simulink model "flatball_hummel_mdl_validation_IC"  (R2021b)
settings: Solver=ode1be  StartTime=0.0  StopTime=30  FixedStep=0.001  MaxStep=0.01  MinStep=0.01  RelTol=1e-3
values from neighbouring files (symbols this model uses):
  amb = evalin( 'base', 'amb')    [flatball_6dof_eqom.m]
  disc = evalin( 'base', 'disc')    [flatball_6dof_eqom.m]    (also in flatball_6dof_init.m = struct; flatball_init_disc_params.m = struct)
  k_launch_F_t_release = 0.60    (= 0.6)    [flatball_6dof_hucker_init.m]
  k_launch_Fx_kd = 2e-2    (= 0.02)    [flatball_6dof_hucker_init.m]
  k_launch_Fx_ki = 15    [flatball_6dof_hucker_init.m]
  k_launch_Fx_kp = 7.5    [flatball_6dof_hucker_init.m]
  k_launch_Fx_sat_hi = 150    [flatball_6dof_hucker_init.m]
  k_launch_Fx_sat_lo = -150    [flatball_6dof_hucker_init.m]
  k_launch_Fx_t_launch_begin = 0.50    (= 0.5)    [flatball_6dof_hucker_init.m]
  k_launch_Fx_t_launch_end = k_launch_F_t_release    (= 0.6)    [flatball_6dof_hucker_init.m]
  k_launch_Fx_tau = 1e-2    (= 0.01)    [flatball_6dof_hucker_init.m]
  k_launch_Fy_kd = k_launch_Fx_kd    (= 0.02)    [flatball_6dof_hucker_init.m]
  k_launch_Fy_ki = k_launch_Fx_ki    (= 15)    [flatball_6dof_hucker_init.m]
  k_launch_Fy_kp = k_launch_Fx_kp    (= 7.5)    [flatball_6dof_hucker_init.m]
  k_launch_Fy_sat_hi = k_launch_Fx_sat_hi    (= 150)    [flatball_6dof_hucker_init.m]
  k_launch_Fy_sat_lo = k_launch_Fx_sat_lo    (= -150)    [flatball_6dof_hucker_init.m]
  k_launch_Fy_t_launch_begin = 0.50    (= 0.5)    [flatball_6dof_hucker_init.m]
  k_launch_Fy_t_launch_end = k_launch_F_t_release    (= 0.6)    [flatball_6dof_hucker_init.m]
  k_launch_Fy_tau = 1e-2    (= 0.01)    [flatball_6dof_hucker_init.m]
  k_launch_Fz_kd = 2.5    [flatball_6dof_hucker_init.m]
  k_launch_Fz_ki = 50    [flatball_6dof_hucker_init.m]
  k_launch_Fz_kp = 20    [flatball_6dof_hucker_init.m]
  k_launch_Fz_sat_hi = 25    [flatball_6dof_hucker_init.m]
  k_launch_Fz_sat_lo = -25    [flatball_6dof_hucker_init.m]
  k_launch_Fz_t_launch_begin = 0.10    (= 0.1)    [flatball_6dof_hucker_init.m]
  k_launch_Fz_t_launch_end = k_launch_F_t_release    (= 0.6)    [flatball_6dof_hucker_init.m]
  k_launch_Fz_tau = 1e-2    (= 0.01)    [flatball_6dof_hucker_init.m]
  k_launch_M_t_release = 0.60    (= 0.6)    [flatball_6dof_hucker_init.m]
  k_launch_Mx_kd = 0.125    [flatball_6dof_hucker_init.m]
  k_launch_Mx_ki = 1.125    [flatball_6dof_hucker_init.m]
  k_launch_Mx_kp = 3.5    [flatball_6dof_hucker_init.m]
  k_launch_Mx_sat_hi = 2.5    [flatball_6dof_hucker_init.m]
  k_launch_Mx_sat_lo = -2.5    [flatball_6dof_hucker_init.m]
  k_launch_Mx_t_launch_begin = 0.30    (= 0.3)    [flatball_6dof_hucker_init.m]
  k_launch_Mx_t_launch_end = k_launch_M_t_release    (= 0.6)    [flatball_6dof_hucker_init.m]
  k_launch_Mx_tau = 1e-2    (= 0.01)    [flatball_6dof_hucker_init.m]
  k_launch_My_kd = 0.1125    [flatball_6dof_hucker_init.m]
  k_launch_My_ki = 5.5    [flatball_6dof_hucker_init.m]
  k_launch_My_kp = 4.25    [flatball_6dof_hucker_init.m]
  k_launch_My_sat_hi = 2.5    [flatball_6dof_hucker_init.m]
  k_launch_My_sat_lo = -2.5    [flatball_6dof_hucker_init.m]
  k_launch_My_t_launch_begin = 0.40    (= 0.4)    [flatball_6dof_hucker_init.m]
  k_launch_My_t_launch_end = k_launch_M_t_release    (= 0.6)    [flatball_6dof_hucker_init.m]
  k_launch_My_tau = 1e-2    (= 0.01)    [flatball_6dof_hucker_init.m]
  k_launch_Mz_kd = 1e-8    (= 1e-08)    [flatball_6dof_hucker_init.m]
  k_launch_Mz_ki = 0.2575    [flatball_6dof_hucker_init.m]
  k_launch_Mz_kp = 0.25    [flatball_6dof_hucker_init.m]
  k_launch_Mz_sat_hi = 7.5    [flatball_6dof_hucker_init.m]
  k_launch_Mz_sat_lo = -7.5    [flatball_6dof_hucker_init.m]
  k_launch_Mz_t_launch_begin = 0.20    (= 0.2)    [flatball_6dof_hucker_init.m]
  k_launch_Mz_t_launch_end = k_launch_M_t_release    (= 0.6)    [flatball_6dof_hucker_init.m]
  k_launch_Mz_tau = 1e-2    (= 0.01)    [flatball_6dof_hucker_init.m]
  X0_crowther_f2302 = [      -0.90 -0.63 -0.91,  4.48 12.52 1.84,      -0.07 0.21 5.03,    -26.25 -5.19 52.85]    [hummel_thesis_mdl_validation.m]
  X0_desired = X0_crowther_f2302    [hummel_thesis_mdl_validation.m]
  X0_hummel_f2302 = [      -0.90 -0.63 -0.91,  13.42 -0.41 0.001,      -0.07 0.21 5.03,    -14.94 -1.48 54.25]    [hummel_thesis_mdl_validation.m]
libraries: slpidlib x6, simulink x2, aerolibanim x2, aerolibnav x2, matrix_library x2, mspfiltlib x1
(part 3 of 3)

== matlab function flatball_hummel_mdl_validation_IC/calc-M/q-inf/vector-norm ==
  data: vec input; norm output
function norm = fcn( vec)

norm = sqrt( vec(1)*vec(1) + vec(2)*vec(2) + vec(3)*vec(3));

== matlab function flatball_hummel_mdl_validation_IC/rotations/X-to-T_c_N ==
  data: X input; T_c_N output
function T_c_N  = f( X)
%% internal states
phi = X(7); theta = X(8);

%% helper variables
sin_theta = sin( theta);
cos_theta = cos( theta);
sin_phi = sin( phi);
cos_phi = cos(phi);

T_c_N = [
    cos_theta sin_theta*sin_phi -sin_theta*cos_phi;
    0 cos_phi sin_phi;
    sin_theta -cos_theta*sin_phi cos_theta*cos_phi
    ];

== matlab function flatball_hummel_mdl_validation_IC/lab/helpers/Subsystem1/transformation-matrices/Ta ==
  data: TH input; M output
function M  = Ta( TH)
% transformation matrix
%
phi = TH(1); theta = TH(2); psi = TH(3);

cos_theta = cos( theta);
cos_phi = cos( phi);
cos_psi = cos( psi);
sin_phi = sin( phi);
sin_theta = sin( theta);
sin_psi = sin( psi);

M = [ ...
    cos_theta*cos_psi sin_phi*sin_theta*cos_phi-cos_phi*sin_psi cos_phi*sin_theta*cos_psi+sin_phi*sin_psi;
    cos_theta*sin_psi sin_phi*sin_theta*sin_psi+cos_phi*cos_psi cos_phi*sin_theta*sin_psi-sin_phi*cos_psi;
    -sin_theta sin_phi*cos_theta cos_phi*cos_theta
    ];

% tan_theta = tan( theta);
% sec_theta = sec( theta);
% transform_r_phi_thea_psi = [
%     1 sin_phi*tan_theta cos_phi*tan_theta
%     0 cos_phi -sin_phi
%     0 sin_phi*sec_theta cos_phi*sec_theta
%     ];

== matlab function flatball_hummel_mdl_validation_IC/rotations/X-to-wD_N_inC ==
  data: X input; wD_N_inC output
function wD_N_inC  = f( X)
%% internal states
theta = X(8);
phidot = X(10); thetadot = X(11); gammadot = X(12);

%% helper variables
sin_theta = sin( theta);
cos_theta = cos( theta);

wD_N_inC = [phidot*cos_theta thetadot phidot*sin_theta+gammadot];

== matlab function flatball_hummel_mdl_validation_IC/lab/wrk/flatball_6dof ==
  data: X input; Xdot output; lift output; drag output; alpha output; AdvR output; E_trans output; E_rot output
function [Xdot, lift, drag, alpha, AdvR, E_trans, E_rot]  = flatball_6dof_eom( X)
% flatball equations of motion - NED (north-east-down) configuration
%

%% internal states
x = X(1); y = X(2); z = X(3);
xdot = X(4); ydot = X(5); zdot = X(6);

phi = X(7); theta = X(8); gamma = X(9);
phidot = X(10); thetadot = X(11); gammadot = X(12);

Xdot = zeros(1,12);

%% define ambient parameters
amb.g = 9.81; % m/s^2
amb.rho = 1.23; % Kg/m^3

%% define non-aerodynamic parameters
disc = struct;
disc.m = 0.175; % Kg
disc.A = 0.057; % m^2
disc.d = 2*sqrt(0.057/pi); % 2*sqrt(disc.A/pi); % diameter
disc.Ia = 0.002352; % moment of inertia about the spinning axis
disc.Id = 0.001219; % moment of inertia about the planar axis'

disc.alpha0 = -4 * pi/180.0;

%% THE THREE ESTIMATED COEFFICIENTS
disc.CMq= -1.44E-02;
disc.CRp =-1.25E-02;
disc.CNr = -3.41E-05; % long flight f2302

%% THE seven COEFFICIENTS estimated from three flights
disc.CL0= 0.3331;
disc.CLa= 1.9124;
disc.CD0= 0.1769;
disc.CDa= 0.685;
disc.CM0= -0.0821;
disc.CMa= 0.4338;
disc.CRr= 0.00171; % for nondimensionalization = sqrt(d/g), magnitude of CRr changes

%% CL =[ rad CL deg]
disc.CL_data=[ -0.1745 -0.2250 -10; ...
-0.05236 0 -3; ...
0 0.150 0; ...
0.08727 0.4500 5; ...
0.17453 0.7250 10; ...
0.26180 0.9750 15; ...
0.34907 1.2000 20; ...
0.43633 1.4500 25; ...
0.52360 1.6750 30];

%% CD =[ rad CD deg]
disc.CD_data=[ -0.1745 0.1500 -10; ...
-0.05236 0.0800 -3; ...
0 0.1000 0; ...
0.08727 0.1500 5; ...
0.1745 0.2600 10; ...
0.26180 0.3900 15; ...
0.3491 0.5700 20; ...
0.4363 0.7500 25; ...
0.5236 0.9200 30];

%% CM =[ rad CM deg]
disc.CM_data=[-0.174532925 -0.0380 -10; ...
-0.087266463 -0.0220 -5; ...
-0.052359878 -0.0140 -3; ...
0 -0.0060 0; ...
0.052359878 -0.0060 3; ...
0.104719755 -0.0020 6; ...
0.157079633 0.0000 9; ...
0.20943951 0.0100 12; ...
0.261799388 0.0220 15; ...
0.34906585 0.0440 20; ...
0.401425728 0.0600 23; ...
0.453785606 0.0840 26; ...
0.523598776 0.1100 30];

%% helper variables
cos_theta = cos( theta);
cos_phi = cos( phi);
cos_psi = cos( psi);
sin_phi = sin( phi);
sin_theta = sin( theta);
sin_psi = sin( psi);
tan_theta = tan( theta);
sec_theta = sec( theta);

transform_a_phi_theta_psi = [ ...
    cos_theta*cos_psi sin_phi*sin_theta*cos_phi-cos_phi*sin_psi cos_phi*sin_theta*cos_psi+sin_phi*sin_psi;
    cos_theta*sin_psi sin_phi*sin_theta*sin_psi+cos_phi*cos_psi cos_phi*sin_theta*sin_psi-sin_phi*cos_psi;
    -sin_theta sin_phi*cos_theta cos_phi*cos_theta
    ];
transform_r_phi_thea_psi = [
    1 sin_phi*tan_theta cos_phi*tan_theta
    0 cos_phi -sin_phi
    0 sin_phi*sec_theta cos_phi*sec_theta
    ];
% c1 = T_c_N(1,:);
% c2 = T_c_N(2,:);
c3 = T_c_N(3,:);

%% aerodynamic forces and moments in N reference frame
vel = [xdot ydot zdot];
vmag = norm( vel);
vc3 = dot( vel, c3);
v_N = [ vel - vc3*c3];
Adp = 0.5 * disc.A * amb.rho * vmag*vmag;
uvel = vel / vmag;
uv_N = v_N / norm( v_N);
u_lat = cross( c3, uv_N);

wD_N_inC = [phidot*cos_theta thetadot phidot*sin_theta+gammadot];
wD_N_inN = T_c_N' * wD_N_inC';

w_v_N = dot( wD_N_inN, uv_N);
w_lat = dot( wD_N_inN, u_lat);
w_spin = dot( wD_N_inN, c3);

alpha = atan( vc3 / norm( v_N)); % angle of attack
AdvR = disc.d * w_spin / 2 / vmag; % advance ratio
E_trans = 0.5 * disc.m * vmag*vmag; % translational energy
E_rot = 0.5 * disc.Ia * gammadot*gammadot; % rotational energy

%% coefficients - f(alpha)
% dalpha = alpha - disc.alpha0;
% Cl = disc.CL0 + disc.CLa * alpha;
% CD = disc.CD0 + disc.CDa * dalpha*dalpha;
% CM = disc.CM0 + disc.CMa * alpha;
% Mv_N = Adp * disc.d * (sqrt(disc.d/amb.g)*disc.CRr*w_spin + disc.CRp*w_v_N) * uv_N;

%% coefficients - lookup based
% hacks
k_CL_gain = 1.0; %2.5;
k_CD_gain = 1.0; %1.5;
k_M_gain = 1.0;
k_decay = 0.25;
% hacks

CL = interp1( disc.CL_data(:,1), disc.CL_data(:,2).*k_CL_gain, alpha, 'spline');
CD = interp1( disc.CD_data(:,1), disc.CD_data(:,2).*k_CD_gain, alpha, 'spline');
CM = interp1( disc.CM_data(:,1), disc.CM_data(:,2).*k_M_gain, alpha, 'spline');
% CRr = interp2( disc.CRr_rad, disc.CRr_AdvR, disc.CRr_data, alpha, AdvR,'spline');
Mv_N = Adp * disc.d * ( disc.CRr* + disc.CRp*w_v_N) * uv_N;

%%
lift = CL * Adp;
drag = CD * Adp;
ulift = -cross( uvel, u_lat);
udrag = -uvel;
Faero = lift*ulift + drag*udrag;
Fg_N = [0 0 disc.m*amb.g]';

F = Faero' + Fg_N;

Mlat = Adp * disc.d * (CM + disc.CMq * w_lat) * u_lat;
Mspin = [0 0 disc.CNr*-1e-5*w_spin];
M = T_c_N * Mv_N' + T_c_N*Mlat' + Mspin';

%%
xdotdot = F(1) / disc.m;
ydotdot = F(2) / disc.m;
zdotdot = F(3) / disc.m;

phidotdot = (M(1) + disc.Id*thetadot*phidot*sin_theta - disc.Ia*thetadot*(phidot*sin_theta+gammadot) + disc.Id*thetadot*phidot*sin_theta)/disc.Id/cos_theta; 
thetadotdot = (M(2) + disc.Ia*phidot*cos_theta*(phidot*sin_theta +gammadot) - disc.Id*phidot*phidot*cos_theta*sin_theta)/disc.Id;
% bug in hummels report?
% gammadotdot = (M(3) - disc.Ia*(phidotdot*sin_theta + thetadot*phidot*cos_theta))/disc.Ia;
% bug in hummels report?
% w/phidotdot term, there is no decay in gammadot
% w/out gammadot term - there is no decay in gammadot
% NOTE: w/it, the decay is too agressive
% FIXME: investigate why this term is necessary for more appropriate
% spindown (based on my data)
gammadotdot = (M(3) - disc.Ia*(k_decay*gammadot*sin_theta + thetadot*phidot*cos_theta))/disc.Ia;

%%
Xdot(1) = xdot;
Xdot(2) = ydot;
Xdot(3) = zdot;

Xdot(4) = xdotdot;
Xdot(5) = ydotdot;
Xdot(6) = zdotdot;

Xdot(7) = phidot;
Xdot(8) = thetadot;
Xdot(9) = gammadot;

Xdot(10) = phidotdot;
Xdot(11) = thetadotdot;
Xdot(12) = gammadotdot;

== matlab function flatball_hummel_mdl_validation_IC/lab/helpers/Subsystem1/transformation-matrices/Tr ==
  data: TH input; M output
function M  = Tr( TH)
% transformation matrix
%
phi = TH(1); theta = TH(2); psi = TH(3);

cos_theta = cos( theta);
cos_phi = cos( phi);
cos_psi = cos( psi);
sin_phi = sin( phi);
sin_theta = sin( theta);
sin_psi = sin( psi);

tan_theta = tan( theta);
sec_theta = sec( theta);

M = [
    1 sin_phi*tan_theta cos_phi*tan_theta
    0 cos_phi -sin_phi
    0 sin_phi*sec_theta cos_phi*sec_theta
    ];

== matlab function flatball_hummel_mdl_validation_IC/lab/helpers/Subsystem/Ta1 ==
  data: phi input; T output; theta input; psi input
function T  = Ta( phi, theta, psi)
% transformation matrix
%

cos_theta = cos( theta);
cos_phi = cos( phi);
cos_psi = cos( psi);
sin_phi = sin( phi);
sin_theta = sin( theta);
sin_psi = sin( psi);

T= [ ...
    cos_theta*cos_psi sin_phi*sin_theta*cos_phi-cos_phi*sin_psi cos_phi*sin_theta*cos_psi+sin_phi*sin_psi;
    cos_theta*sin_psi sin_phi*sin_theta*sin_psi+cos_phi*cos_psi cos_phi*sin_theta*sin_psi-sin_phi*cos_psi;
    -sin_theta sin_phi*cos_theta cos_phi*cos_theta
    ];

% tan_theta = tan( theta);
% sec_theta = sec( theta);
% transform_r_phi_thea_psi = [
%     1 sin_phi*tan_theta cos_phi*tan_theta
%     0 cos_phi -sin_phi
%     0 sin_phi*sec_theta cos_phi*sec_theta
%     ];

== matlab function flatball_hummel_mdl_validation_IC/lab/helpers/Subsystem2/Ta2 ==
  data: phi input; T output; theta input; psi input
function T  = Ta( phi, theta, psi)
% transformation matrix
%

cos_theta = cos( theta);
cos_phi = cos( phi);
cos_psi = cos( psi);
sin_phi = sin( phi);
sin_theta = sin( theta);
sin_psi = sin( psi);

T= [ ...
    cos_theta*cos_psi sin_phi*sin_theta*cos_phi-cos_phi*sin_psi cos_phi*sin_theta*cos_psi+sin_phi*sin_psi;
    cos_theta*sin_psi sin_phi*sin_theta*sin_psi+cos_phi*cos_psi cos_phi*sin_theta*sin_psi-sin_phi*cos_psi;
    -sin_theta sin_phi*cos_theta cos_phi*cos_theta
    ];

% tan_theta = tan( theta);
% sec_theta = sec( theta);
% transform_r_phi_thea_psi = [
%     1 sin_phi*tan_theta cos_phi*tan_theta
%     0 cos_phi -sin_phi
%     0 sin_phi*sec_theta cos_phi*sec_theta
%     ];

== matlab function flatball_hummel_mdl_validation_IC/lab/helpers/Subsystem1/w_ ==
  data: THdot input; M output
function M  = w_( THdot)
% transformation matrix
%
p = THdot(1); q = THdot(2); r = THdot(3);

M = [ ...
    0 -r q;
    r 0 -p;
    -q p 0
    ];

== matlab function flatball_hummel_mdl_validation_IC/lab/helpers/Subsystem/zero-side-slip-angle ==
  data: Xdot input; beta output
function beta  = f( Xdot)
% calculate side-slip angle

beta = atan( Xdot(2) / Xdot(1));
